simulink model "power_compensated"  (Simulink 6.0)
settings: Solver=ode15s  SolverMode=SingleTasking  StartTime=0.0  StopTime=0.4  RelTol=1e-4
libraries: powerlib x31
settings Model: Creator=patrice  LastModifiedBy=batserve  ExtModeTrigMode=oneshot  ExtModeArmWhenConnect=off  ExtModeAutoUpdateStatusClock=off
settings DataIOCC: ExternalInput=[]  LimitDataPoints=off  SaveOutput=off  SignalLoggingName=sigsOut
settings OptimizationCC: BlockReduction=off  BooleanDataType=off
settings DebuggingCC: AlgebraicLoopMsg=none  CheckExecutionContextPreStartOutputMsg=on  CheckExecutionContextRuntimeOutputMsg=on  SolverPrmCheckMsg=none
settings HardwareCC: TargetUnknown=on
settings RTWCC: TemplateMakefile=grt_unix.tmf

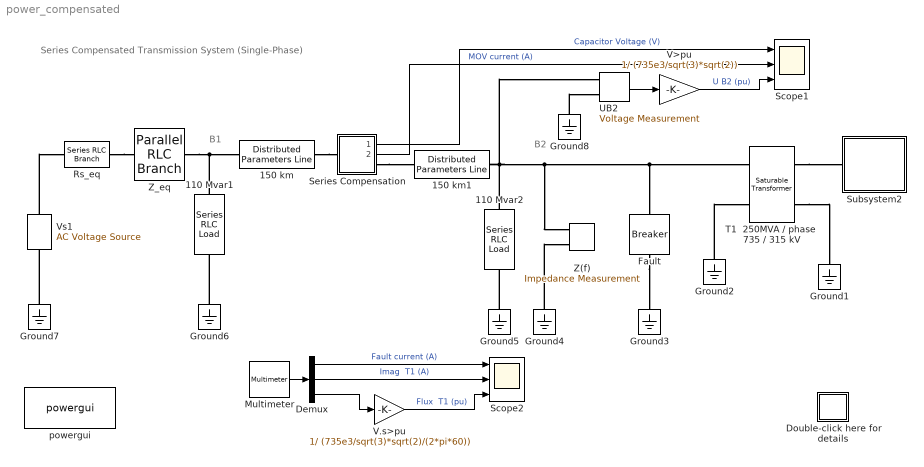
== system power_compensated ==
  note: Series Compensated Transmission System
      | (Single-Phase)
  note: B1
  note: B2
  110 Mvar1 : powerlib/Elements/Series RLC Load  Orientation=up  PhysicalDomain=powersysdomain  SubClassName=unknown  LeftPortType=p1  RightPortType=p1  LConnTagsString=a  RConnTagsString=__new0  NominalVoltage=735000/sqrt(3)  NominalFrequency=60  ActivePower=110e6/300  InductivePower=110e6  CapacitivePower=0  Measurements=None
  110 Mvar2 : powerlib/Elements/Series RLC Load  Orientation=up  PhysicalDomain=powersysdomain  SubClassName=unknown  LeftPortType=p1  RightPortType=p1  LConnTagsString=a  RConnTagsString=__new0  NominalVoltage=735000/sqrt(3)  NominalFrequency=60  ActivePower=110e6/300  InductivePower=110e6  CapacitivePower=0  Measurements=None
  150 km : powerlib/Elements/Distributed Parameters Line  Phases=1  Frequency=60  Resistance=0.011  Inductance=0.8674e-03  Capacitance=13.41e-09  Length=150  x1=[0 0 0 0; 0.0001244 0 0 0; 0.0002488 0 0 0; 0.0003733 0 0 0; 0.0004977 0 0 0; 0.0006221 0 0 0]  x2=[0 0 0 0; 0.0001244 0 0 0; 0.0002488 0 0 0; 0.0003733 0 0 0; 0.0004977 0 0 0; 0.0006221 0 0 0]  x3=[0 0 0 0; 0.0001244 0 0 0; 0.0002488 0 0 0; 0.0003733 0 0 0; 0.0004977 0 0 0; 0.0006221 0 0 0]  x4=[0 0 0 0; 0.0001244 0 0 0; 0.0002488 0 0 0; 0.0003733 0 0 0; 0.0004977 0 0 0; 0.0006221 0 0 0]  x5=0  Measurements=None
      settings: AttributesFormatString=\n
  150 km1 : powerlib/Elements/Distributed Parameters Line  Phases=1  Frequency=60  Resistance=0.011  Inductance=0.8674e-03  Capacitance=13.41e-09  Length=150  x1=[0 0 0 0; 0.0001244 0 0 0; 0.0002488 0 0 0; 0.0003733 0 0 0; 0.0004977 0 0 0; 0.0006221 0 0 0]  x2=[0 0 0 0; 0.0001244 0 0 0; 0.0002488 0 0 0; 0.0003733 0 0 0; 0.0004977 0 0 0; 0.0006221 0 0 0]  x3=[0 0 0 0; 0.0001244 0 0 0; 0.0002488 0 0 0; 0.0003733 0 0 0; 0.0004977 0 0 0; 0.0006221 0 0 0]  x4=[0 0 0 0; 0.0001244 0 0 0; 0.0002488 0 0 0; 0.0003733 0 0 0; 0.0004977 0 0 0; 0.0006221 0 0 0]  x5=0  Measurements=None
      settings: AttributesFormatString=\n
  Demux : Demux  Outputs=3
  Double-click here for details : Subsystem
      mask Display: disp('?')
  Fault : powerlib/Elements/Breaker  Orientation=down  BreakerResistance=0.01  InitialState=0  SnubberResistance=inf  SnubberCapacitance=0  SwitchingTimes="[ 3/60  9/60 ]"  External=off  Measurements=Branch current
      settings: AttributesFormatString=\n
  Ground{1..8} (8 alike) : powerlib/Elements/Ground  Orientation=down  PhysicalDomain=powersysdomain  SubClassName=unknown  LeftPortType=p1  RightPortType=p1  LConnTagsString=a
  Multimeter : powerlib/Measurements/Multimeter  Tag=PoWeRsYsTeMmEaSuReMeNt  PhasorSimulation=off  OutputType=Magnitude  sel=[1 2 3]  L=3  Gain=[1 1 1]  yselected="{'Ib: Fault','Imag: T1  250MVA // phase  735 // 315 kV','Flux: T1  250MVA // phase  735 // 315 kV'};"  PSBOutputType=1  PSBequivalent=0  AxesSetting=[0,0.1,-100,100]  Display=0  SavedBlockNames={}
      settings: AttributesFormatString=\n
  Rs_eq : powerlib/Elements/Series RLC Branch  PhysicalDomain=powersysdomain  SubClassName=unknown  LeftPortType=p1  RightPortType=p1  LConnTagsString=__new0  RConnTagsString=__new0  Resistance=2  Inductance=0  Capacitance=inf  Measurements=None
  Scope1 : Scope  NumInputPorts=3
      settings: DeleteFcn=simscope BlockIsBeingDestroyed  PostSaveFcn=simscope Save  TimeRange=0.4  YMin=-400000~-10000~-2  YMax=400000~10000~2  DataFormat=Array  MaxDataPoints=100000000
  Scope2 : Scope  NumInputPorts=3
      settings: DeleteFcn=simscope BlockIsBeingDestroyed  PostSaveFcn=simscope Save  TimeRange=0.4  YMin=-10000~-2000~-2  YMax=10000~1000~2  DataFormat=Array  MaxDataPoints=100000000
  Series Compensation : Subsystem
      mask Display: plot(0,0,100,100,[10 40],[50 50], [40 40],[40 60],[60 60],[40 60], [60 90],[50 50])
  Subsystem2 : Subsystem
      mask Display: disp('315 kV\nEquivalent')
  T1  250MVA / phase  735 / 315 kV : powerlib/Elements/Saturable Transformer  NominalPower=[750e6/3,60]  Winding1=[735000/sqrt(3), 0.001 ,0.15]  Winding2=[315000/sqrt(3), 0.001,0]  ThreeWindings=off  Winding3=[315000/sqrt(3), 0.001,0]  Saturation=[0 0 ; 0.0012 1.2; 1.0 1.45 ]  CoreLoss=[1000]  Hysteresis=off  DataFile='hysteresis'  Measurements=Flux and magnetization current ( Imag )  InitialFlux=0  TransfoNumber=1
      settings: AttributesFormatString=\n
  UB2 : powerlib/Measurements/Voltage Measurement  Tag=PoWeRsYsTeMmEaSuReMeNt  PhasorSimulation=off  OutputType=Magnitude  PSBequivalent=0
  V.s>pu : Gain  Gain=1/ (735e3/sqrt(3)*sqrt(2)/(2*pi*60))  SaturateOnIntegerOverflow=on
  V>pu : Gain  Gain=1/ (735e3/sqrt(3)*sqrt(2))  SaturateOnIntegerOverflow=on
  Vs1 : powerlib/Electrical Sources/AC Voltage Source  Description=source block  Orientation=up  Amplitude=735000/sqrt(3)*sqrt(2)  Phase=0  Frequency=60  SampleTime=0  Measurements=None
      settings: AttributesFormatString=\n
  Z(f) : powerlib/Measurements/Impedance Measurement  PhysicalDomain=powersysdomain  SubClassName=unknown  LeftPortType=p1  RightPortType=p1  LConnTagsString=+|-  Factor=1
      settings: AttributesFormatString=\n
  Z_eq : powerlib/Elements/Parallel RLC Branch  PhysicalDomain=powersysdomain  SubClassName=unknown  LeftPortType=p1  RightPortType=p1  LConnTagsString=a  RConnTagsString=__new0  Resistance=180.1  Inductance=.026525  Capacitance=117.84e-06  Measurements=None
  powergui : powerlib/powergui  Priority=2  Frange=0:500  Ylog=off  Xlog=off  save=off  variable=ZData  ZoomFFT=on  StartTime=0.0  cycles=2  DisplayStyle=off  fundamental=60  FreqAxis=off  MaxFrequency=1000  frequencyindice=1  frequencyindicesteady=1  RmsSteady=1  display=off  Ts=0  methode=off  frequency=60  echomessages=off
  wires:
  V>pu/1 -> Scope1/3  "U B2 (pu)"
  Demux/3 -> V.s>pu/1
  Demux/1 -> Scope2/1  "Fault current (A)"
  V.s>pu/1 -> Scope2/3  "Flux  T1 (pu)"
  Demux/2 -> Scope2/2  "Imag  T1 (A)"
  Multimeter/1 -> Demux/1
  UB2/1 -> V>pu/1
  Series Compensation/1(V_Cs) -> Scope1/1  "Capacitor Voltage (V)"
  Series Compensation/2(I_MOV) -> Scope1/2  "MOV current (A)"
  connections:
  T1  250MVA / phase  735 / 315 kV/RConn2 -- Ground1/LConn1
  Ground2/LConn1 -- T1  250MVA / phase  735 / 315 kV/LConn2
  Fault/RConn1 -- Ground3/LConn1
  Ground6/LConn1 -- 110 Mvar1/LConn1
  Ground7/LConn1 -- Vs1/LConn1
  Vs1/RConn1 -- Rs_eq/LConn1
  Z_eq/RConn1 -- 150 km/LConn1 -- 110 Mvar1/RConn1
  Ground5/LConn1 -- 110 Mvar2/LConn1
  T1  250MVA / phase  735 / 315 kV/RConn1 -- Subsystem2/LConn1
  Ground4/LConn1 -- Z(f)/LConn2
  150 km/RConn1 -- Series Compensation/LConn1
  Rs_eq/RConn1 -- Z_eq/LConn1
  150 km1/RConn1 -- 110 Mvar2/RConn1 -- UB2/LConn1 -- T1  250MVA / phase  735 / 315 kV/LConn1 -- Fault/LConn1 -- Z(f)/LConn1
  Ground8/LConn1 -- UB2/LConn2
  Series Compensation/RConn1 -- 150 km1/LConn1

== system power_compensated/Double-click here for details ==
  note: Demonstration
  note: This demonstration ilustrates frequency-domain and time-domain analysis of
      | a series-compensated  transmission system
  note: Circuit Description
  note: A 735 kV, 300 km  line is used to  transmit power from bus B1 (735 kV equivalent system) to bus B2 (315 kV equivalent).
      | In order to simplify, only one phase of the system has been represented.
      | (A detailed simulation of  a three-phase series compensated network is presented in demo power_3phseries and explained in the case studies
      | section of the user's manual.)
      |
      | In order to increase the transmission capacity, the line is series compensated at its center by a capacitor representing 40% of the line reactance.
      | The line is also shunt compensated at both ends by a 330 Mvar shunt reactance (110 Mvar /phase).
      | Open the  Series Compensation subsystem. Notice that the series capacitor is protected by a metal oxide varistor (MOV) simulated by the Surge Arrester block.
      | The 250 MVA, 735 kV / 315 kV transformer is a Saturable Transformer block simulating one phase of the three-phase 750 MVA transformer.
      | A  Multimeter block is used to monitor the fault current as well as the flux and magnetizing current of the transformer.
  note: You now study the transient performance of this circuit when a 6-cycle fault is applied at node B2.
      | Fault is simulated by the Breaker block. Switching times are defined in the Breaker block menu (closing at t = 3 cycles and opening at t = 9 cycles).
  note: Start the simulatiom and observe waveforms on the two Scopes.
      | At t = 3 cycles, a line-to-ground fault is applied and the fault current reaches 10 kA (trace 1 of Scope2).
      | During the fault, the MOV conducts at every half cycle (trace 2 of Scope1) and the voltage across the capacitor (trace 1 of Scope1)  is limited to 263 kV.
      | At t = 9 cycles, the fault is cleared. The 15 Hz mode is clearly seen on the capacitor voltage (trace 1 of Scope1) and bus B2 voltage (trace 3 of Scope1).
      | During fault the flux in the transformer is trapped to around 1 pu. At fault clearing  the flux offset and 15 Hz component cause transformer
      | saturation (flux > 1.2 pu, trace 3 of Scope2), producing magnetizing current pulses (trace 2 of Scope2).
  note: Frequency Analysis
  note: Time Domain Simulation - Fault at Bus B2
  note: In order to understand the transient behavior of this series-compensated network, a frequency analysis is first preformed by measuring the Impedance at node B2.
      | This  measurement is performed by the Impedance Measurement block connected at node B2.
      | Open the Powergui and in the Tools menu select 'Impedance vs Frequency Mesurement'. Click on Display to compute and display the impedance for the 0 - 500 Hz range.
      | The impedance curves show two main parallel resonances (impedance maxima and phase inversion), corresponding to 15 Hz and 300 Hz modes.
      | The 15 Hz mode is due to a parallel resonance of the series capacitance and the two shunt reactances.
      | The 300 Hz mode is  mainly due to resonance of shunt line capacitance and series reactance of the transmission system.
      | These two modes are likely to be excited at fault clearing.
  note: G. Sybille (Hydro-Quebec)

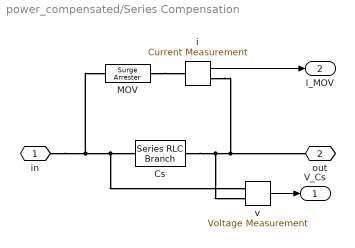
== system power_compensated/Series Compensation ==
  Cs : powerlib/Elements/Series RLC Branch  PhysicalDomain=powersysdomain  SubClassName=unknown  LeftPortType=p1  RightPortType=p1  LConnTagsString=__new0  RConnTagsString=__new0  Resistance=0  Inductance=0  Capacitance=67.6e-6  Measurements=None
  MOV : powerlib/Elements/Surge Arrester  ProtectionVoltage=277e+03  Columns=30  ReferenceCurrent=500  Segment1=[.955 50]  Segment2=[1.0 25]  Segment3=[.9915 16.5]  Measurements=None  MoreParameters=off  BreakLoop=on
      settings: AttributesFormatString=\n
  i : powerlib/Measurements/Current Measurement  Tag=PoWeRsYsTeMmEaSuReMeNt  PhasorSimulation=off  OutputType=Magnitude  PSBequivalent=0
  v : powerlib/Measurements/Voltage Measurement  Tag=PoWeRsYsTeMmEaSuReMeNt  PhasorSimulation=off  OutputType=Magnitude  PSBequivalent=0
  in : PMIOPort  Port=1  Side=Left
  out : PMIOPort  Orientation=left  Port=2  Side=Right
  V_Cs : Outport
  I_MOV : Outport  Port=2
  wires:
  i/1 -> I_MOV/1
  v/1 -> V_Cs/1
  connections:
  in/RConn1 -- Cs/LConn1 -- v/LConn1 -- MOV/LConn1
  MOV/RConn1 -- i/LConn1
  Cs/RConn1 -- out/RConn1 -- i/RConn1 -- v/LConn2

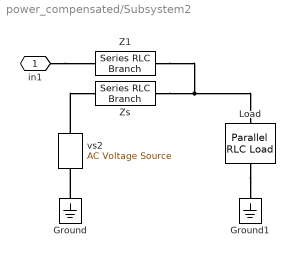
== system power_compensated/Subsystem2 ==
  Ground : powerlib/Elements/Ground  Orientation=down  PhysicalDomain=powersysdomain  SubClassName=unknown  LeftPortType=p1  RightPortType=p1  LConnTagsString=a
  Ground1 : powerlib/Elements/Ground  Orientation=down  PhysicalDomain=powersysdomain  SubClassName=unknown  LeftPortType=p1  RightPortType=p1  LConnTagsString=a
  Load : powerlib/Elements/Parallel RLC Load  Orientation=down  PhysicalDomain=powersysdomain  SubClassName=unknown  LeftPortType=p1  RightPortType=p1  LConnTagsString=a  RConnTagsString=__new0  NominalVoltage=315000/sqrt(3)  NominalFrequency=60  ActivePower=200e6  InductivePower=0  CapacitivePower=50e6  Measurements=None
      settings: AttributesFormatString=\n
  Z1 : powerlib/Elements/Series RLC Branch  PhysicalDomain=powersysdomain  SubClassName=unknown  LeftPortType=p1  RightPortType=p1  LConnTagsString=__new0  RConnTagsString=__new0  Resistance=0.734  Inductance=0.02085  Capacitance=inf  Measurements=None
  Zs : powerlib/Elements/Series RLC Branch  PhysicalDomain=powersysdomain  SubClassName=unknown  LeftPortType=p1  RightPortType=p1  LConnTagsString=__new0  RConnTagsString=__new0  Resistance=11.0  Inductance=0.2925  Capacitance=inf  Measurements=None
  vs2 : powerlib/Electrical Sources/AC Voltage Source  Description=source block  Orientation=up  Amplitude=315000/sqrt(3)*sqrt(2)  Phase=20  Frequency=60  SampleTime=0  Measurements=None
      settings: AttributesFormatString=\n
  in1 : PMIOPort  Port=1  Side=Left
  connections:
  Load/RConn1 -- Ground1/LConn1
  Z1/RConn1 -- Load/LConn1 -- Zs/RConn1
  in1/RConn1 -- Z1/LConn1
  vs2/RConn1 -- Zs/LConn1
  Ground/LConn1 -- vs2/LConn1
